simulink model "RotationTesting"  (R2023a)
settings: Solver=FixedStepAuto  StartTime=0.0  StopTime=10.0  RelTol=1e-3
undefined symbols (not defined in the file or in its folder): InputPWM, WheelSpeed
libraries: arduinolib x8, mobileRoboticsTrainingLib x1
settings Model: ExtModeTrigDuration=2  Creator=siyan  LastModifiedBy=siyan
settings OptimizationCC: EnhancedBackFolding=on  PassReuseOutputArgsAs=Individual arguments  ZeroExternalMemoryAtStartup=off  ZeroInternalMemoryAtStartup=off  MaxStackSize=64  OptimizeBlockOrder=speed  DifferentSizesBufferReuse=on  OptimizationCustomize=off  EfficientTunableParamExpr=on
settings DebuggingCC: ParameterTunabilityLossMsg=error
settings HardwareCC: ProdBitPerPointer=32  ProdBitPerSizeT=32  ProdBitPerPtrDiffT=32  ProdLargestAtomicInteger=Long  ProdLargestAtomicFloat=Double  ProdWordSize=32  ProdHWDeviceType=ARM Compatible->ARM Cortex  UseEmbeddedCoderFeatures=off
settings SFSimCC: MATLABDynamicMemAlloc=off
settings RTWCC: Description=Embedded Coder  SystemTargetFile=ert.tlc  HardwareBoard=Arduino Nano 33 IoT  TemplateMakefile=ert_default_tmf  Toolchain=Arduino ARM  BuildConfiguration=Faster Runs
settings CodeAppCC: ForceParamTrailComments=on  IgnoreCustomStorageClasses=off  OperatorAnnotations=on  SimulinkDataObjDesc=on  SFDataObjDesc=on  InsertBlockDesc=on
settings ERTTargetCC: SupportContinuousTime=on  SupportNonInlinedSFcns=on  SupportVariableSizeSignals=on  ExtModeTransport=3  ExtModeStaticAlloc=on  ExtModeAutomaticAllocSize=off  ExtModeStaticAllocSize=8192  ExtModeMexFile=ext_xcp  ExtModeIntrfLevel=Level2 - Open

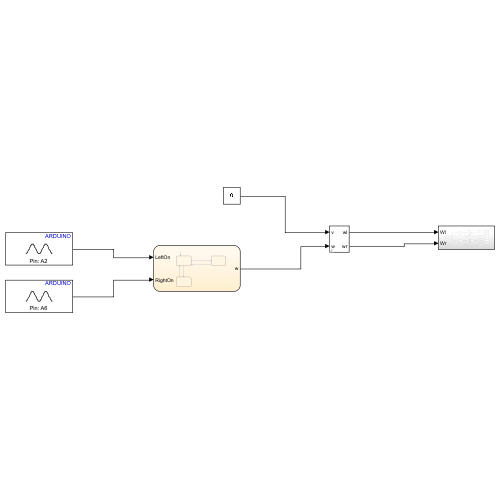
[thumbnail: Simulink's stored preview of the top-level diagram]
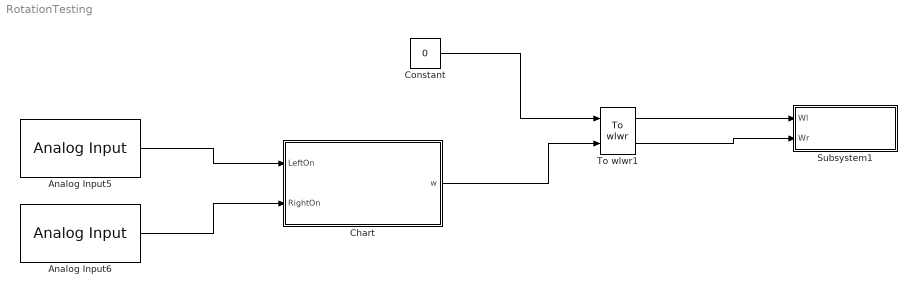
== system RotationTesting ==
  Analog Input5 : arduinolib/Analog Input  pinNumber=2  ReadResultsOnly=off  ConversionTriggerSource=Software  ExternalTriggerType=uint32( 0 )  OutputDataType=uint16  EnableConversionCompleteNotify=off  EnableOuputStatus=off  SampleTime=-1  blockPlatform=arduino
  Analog Input6 : arduinolib/Analog Input  pinNumber=6  ReadResultsOnly=off  ConversionTriggerSource=Software  ExternalTriggerType=uint32( 0 )  OutputDataType=uint16  EnableConversionCompleteNotify=off  EnableOuputStatus=off  SampleTime=-1  blockPlatform=arduino
  Chart : Stateflow chart  TreatAsAtomicUnit=on
  Constant : Constant  Value=0
  Subsystem1 : Subsystem
      settings: LibrarySourceBlock=|
      | hdlsllib/Ports &
      | Subsystems/Subsystem
  To wlwr1 : mobileRoboticsTrainingLib/To wlwr  axleLength=axleLength  wheelR=wheelR
      link override change parameters: Gain=[1 +axleLength/2; 1 -axleLength/2]
  wires:
  To wlwr1/2 -> Subsystem1/2(Wr)
  To wlwr1/1 -> Subsystem1/1(Wl)
  Chart/1(w) -> To wlwr1/2
  Constant/1 -> To wlwr1/1
  Analog Input5/1 -> Chart/1(LeftOn)
  Analog Input6/1 -> Chart/2(RightOn)

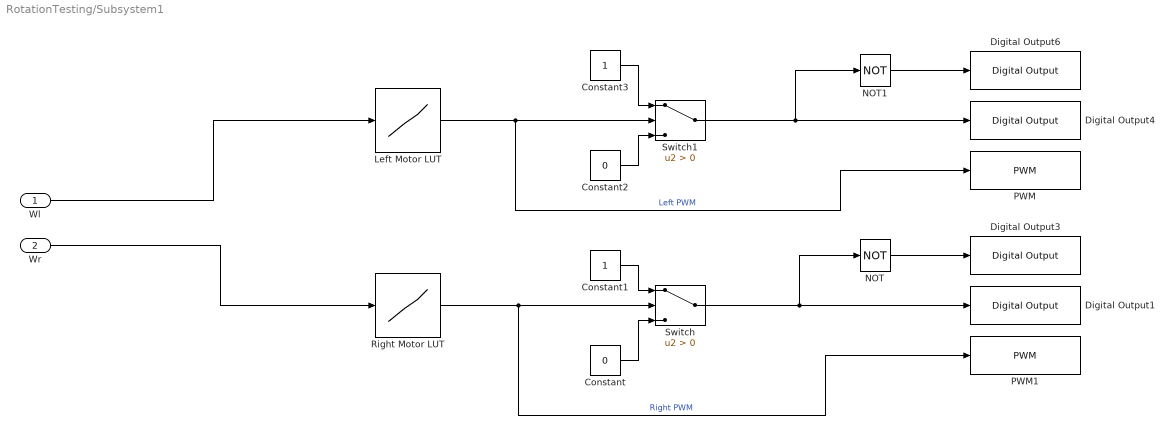
== system RotationTesting/Subsystem1 ==
  Wl : Inport
  Wr : Inport  Port=2
  Constant : Constant  Value=0
  Constant1 : Constant
  Constant2 : Constant  Value=0
  Constant3 : Constant
  Digital Output1 : arduinolib/Digital Output  pinNumber=8  Direction=output  blockPlatform=arduino
  Digital Output3 : arduinolib/Digital Output  pinNumber=11  Direction=output  blockPlatform=arduino
  Digital Output4 : arduinolib/Digital Output  pinNumber=13  Direction=output  blockPlatform=arduino
  Digital Output6 : arduinolib/Digital Output  pinNumber=12  Direction=output  blockPlatform=arduino
  Left Motor LUT : Lookup_n-D  NumberOfTableDimensions=1  BreakpointsForDimension1=WheelSpeed  Table=InputPWM  InterpMethod=Nearest  ExtrapMethod=Clip  InternalRulePriority=Speed  RndMeth=Simplest
  NOT : Logic  Operator=NOT  IconShape=distinctive  AllPortsSameDT=off  OutDataTypeStr=boolean
  NOT1 : Logic  Operator=NOT  IconShape=distinctive  AllPortsSameDT=off  OutDataTypeStr=boolean
  PWM : arduinolib/PWM  pinNumber=9  frequencyType=Default  desiredFrequency=490.2  achievableFrequency=490.2
  PWM1 : arduinolib/PWM  pinNumber=10  frequencyType=Default  desiredFrequency=490.2  achievableFrequency=490.2
  Right Motor LUT : Lookup_n-D  NumberOfTableDimensions=1  BreakpointsForDimension1=WheelSpeed  Table=InputPWM  InterpMethod=Nearest  ExtrapMethod=Clip  InternalRulePriority=Speed  RndMeth=Simplest
  Switch : Switch  Criteria=u2 > Threshold  SaturateOnIntegerOverflow=off  InputSameDT=off
  Switch1 : Switch  Criteria=u2 > Threshold  SaturateOnIntegerOverflow=off  InputSameDT=off
  wires:
  Wr/1 -> Right Motor LUT/1
  Wl/1 -> Left Motor LUT/1
  Right Motor LUT/1 -> PWM1/1, Switch/2  "Right PWM"
  Left Motor LUT/1 -> PWM/1, Switch1/2  "Left PWM"
  NOT1/1 -> Digital Output6/1
  Constant1/1 -> Switch/1
  Constant/1 -> Switch/3
  Constant2/1 -> Switch1/3
  Constant3/1 -> Switch1/1
  Switch/1 -> NOT/1, Digital Output1/1
  Switch1/1 -> NOT1/1, Digital Output4/1
  NOT/1 -> Digital Output3/1

== stateflow chart RotationTesting/Chart ==
  state Pause1
    entry:
    v=0.5
    w=0
  state Left1
    entry:
    v=0.5
    w=2
  state Pause [commented out]
    entry:
    w=0
  state Left [commented out]
    entry:
    w=0.5
  state Right1
    entry:
    v=0.5
    w=-2
  state Right [commented out]
    entry:
    w=-0.5
  (default) -> Pause1
  (default) -> Pause [commented out]
  Pause1 -> Left1 : [after(5,sec)]
  Pause -> Left [commented out] : [RightOn >2]
  Right1 -> Pause1 : [after(5,sec)]
  Left1 -> Right1 : [after(5,sec)]
  Left -> Pause [commented out] : [RightOn < 1]
  Right -> Pause [commented out] : [LeftOn < 1]
  Pause -> Right [commented out] : [LeftOn>2]
  data: w output; LeftOn input; RightOn input
